simulink model "protocol_mc"  (R2021b)
settings: Solver=FixedStepAuto  StartTime=0.0  StopTime=10.0  RelTol=1e-3
settings Model: Creator=marco  LastModifiedBy=angelo
settings ModelReferenceCC: UpdateModelReferenceTargets=IfOutOfDate
settings ConfigComp: DVTestSuiteOptimization=Auto  DVDetectOutOfBounds=on  DVModelReferenceHarness=on

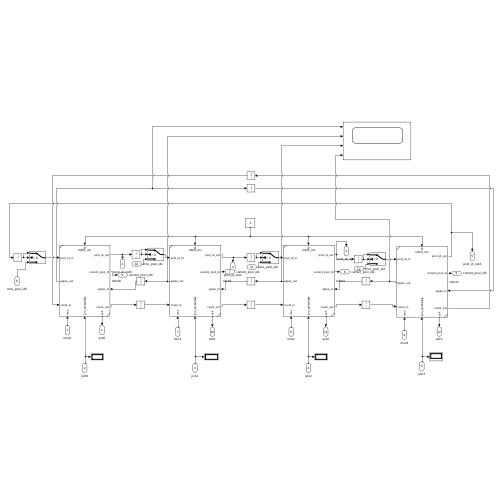
[thumbnail: Simulink's stored preview of the top-level diagram]
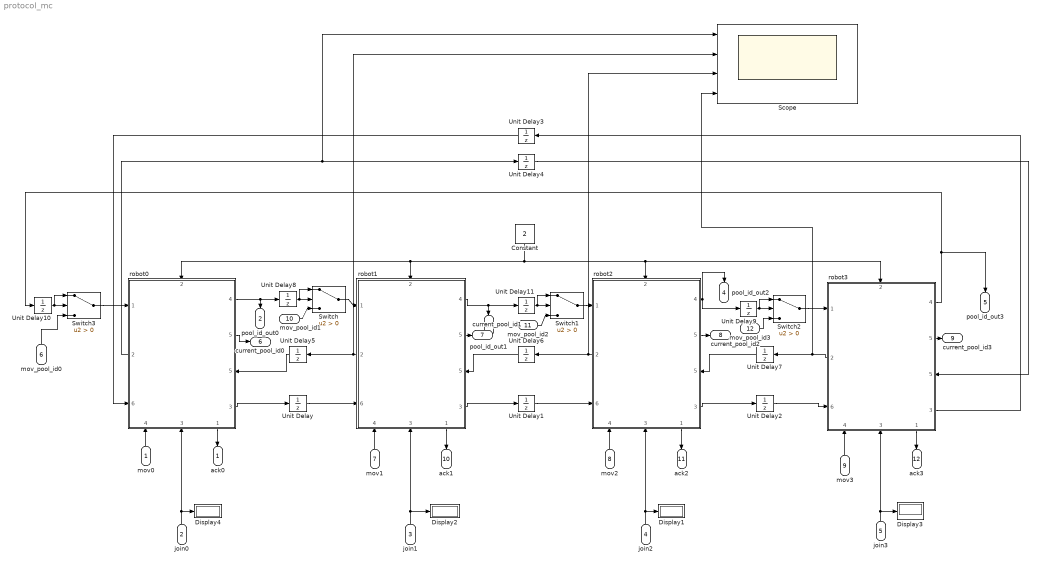
== system protocol_mc ==
  mov0 : Inport
  join0 : Inport  Port=2
  join1 : Inport  Port=3
  join2 : Inport  Port=4
  join3 : Inport  Port=5
  mov_pool_id0 : Inport  Port=6
  mov1 : Inport  Port=7
  mov2 : Inport  Port=8
  mov3 : Inport  Port=9
  mov_pool_id1 : Inport  Port=10
  mov_pool_id2 : Inport  Port=11
  mov_pool_id3 : Inport  Port=12
  Constant : Constant  Value=2
  Display{1..4} (4 alike) : Display
  Scope : Scope  NumInputPorts=4
  Switch{,1..3} (4 alike) : Switch  Criteria=u2 > Threshold
  Unit Delay{,1..11} (12 alike) : UnitDelay  SampleTime=-1  HasFrameUpgradeWarning=on
  robot{0..3} (4 alike) : Subsystem  ReferencedSubsystem=robot_mc
      robot0 settings: PortSchema="{\"entries\":[{\"content\":{\"sides\":[{\"content\":{\"connectorIds\":[\"In1\",\"Out2\",\"In6\"]},\"type\":\"ConnectorPlacement.EquallySpacedRectSide\",\"uuid\":\"c2973ddf-8c1f-4294-82f9-250d4d64bc41\"},{\"content\":{\"connectorIds\":[\"Out4\",\"Out5\",\"In5\",\"Out3\"],\"side\":\"RIGHT\"},\"type\":\"ConnectorPlacement.EquallySpacedRectSide\",\"uuid\":\"34f58778-6b96-4f4c-9fc2-6c1c729063a8\"},{\"content\":{\"connectorIds\":[\"In2\"],\"side\":\"TOP\"},\"type\":\"ConnectorPlacement.EquallySpacedRectSide\",\"uuid\":\"80e910fc-ff47-444b-b672-e337659921ae\"},{\"content\":{\"connectorIds\":[\"In4\",\"In3\",\"Out1\"],\"side\":\"BOTTOM\"},\"type\":\"ConnectorPlacement.EquallySpacedRectSide\",\"uuid\":\"4c5b4a6c-4ee5-43a5-b389-1d5635d4cbda\"}]},\"type\":\"ConnectorPlacement.EquallySpacedConnector\",\"uuid\":\"573bf93a-1f25-4267-812c-06cdd99b033a\"}],\"packageUris\":[\"http://schema.mathworks.com/mf0/Connector/R2020b\"],\"version\":\"1.0\"}"
      robot1 settings: PortSchema="{\"entries\":[{\"content\":{\"sides\":[{\"content\":{\"connectorIds\":[\"In1\",\"Out2\",\"In6\"]},\"type\":\"ConnectorPlacement.EquallySpacedRectSide\",\"uuid\":\"c2973ddf-8c1f-4294-82f9-250d4d64bc41\"},{\"content\":{\"connectorIds\":[\"Out4\",\"Out5\",\"In5\",\"Out3\"],\"side\":\"RIGHT\"},\"type\":\"ConnectorPlacement.EquallySpacedRectSide\",\"uuid\":\"34f58778-6b96-4f4c-9fc2-6c1c729063a8\"},{\"content\":{\"connectorIds\":[\"In2\"],\"side\":\"TOP\"},\"type\":\"ConnectorPlacement.EquallySpacedRectSide\",\"uuid\":\"80e910fc-ff47-444b-b672-e337659921ae\"},{\"content\":{\"connectorIds\":[\"In4\",\"In3\",\"Out1\"],\"side\":\"BOTTOM\"},\"type\":\"ConnectorPlacement.EquallySpacedRectSide\",\"uuid\":\"e4e016b7-b76e-4e62-a0db-89e9df8dea8e\"}]},\"type\":\"ConnectorPlacement.EquallySpacedConnector\",\"uuid\":\"573bf93a-1f25-4267-812c-06cdd99b033a\"}],\"packageUris\":[\"http://schema.mathworks.com/mf0/Connector/R2020b\"],\"version\":\"1.0\"}"
      robot2 settings: PortSchema="{\"entries\":[{\"content\":{\"sides\":[{\"content\":{\"connectorIds\":[\"In1\",\"Out2\",\"In6\"]},\"type\":\"ConnectorPlacement.EquallySpacedRectSide\",\"uuid\":\"c2973ddf-8c1f-4294-82f9-250d4d64bc41\"},{\"content\":{\"connectorIds\":[\"Out4\",\"Out5\",\"In5\",\"Out3\"],\"side\":\"RIGHT\"},\"type\":\"ConnectorPlacement.EquallySpacedRectSide\",\"uuid\":\"34f58778-6b96-4f4c-9fc2-6c1c729063a8\"},{\"content\":{\"connectorIds\":[\"In2\"],\"side\":\"TOP\"},\"type\":\"ConnectorPlacement.EquallySpacedRectSide\",\"uuid\":\"80e910fc-ff47-444b-b672-e337659921ae\"},{\"content\":{\"connectorIds\":[\"In4\",\"In3\",\"Out1\"],\"side\":\"BOTTOM\"},\"type\":\"ConnectorPlacement.EquallySpacedRectSide\",\"uuid\":\"2cd792df-4aad-4f2e-80f9-e48174994b0d\"}]},\"type\":\"ConnectorPlacement.EquallySpacedConnector\",\"uuid\":\"573bf93a-1f25-4267-812c-06cdd99b033a\"}],\"packageUris\":[\"http://schema.mathworks.com/mf0/Connector/R2020b\"],\"version\":\"1.0\"}"
      robot3 settings: PortSchema="{\"entries\":[{\"content\":{\"sides\":[{\"content\":{\"connectorIds\":[\"In1\",\"Out2\",\"In6\"]},\"type\":\"ConnectorPlacement.EquallySpacedRectSide\",\"uuid\":\"c2973ddf-8c1f-4294-82f9-250d4d64bc41\"},{\"content\":{\"connectorIds\":[\"Out4\",\"Out5\",\"In5\",\"Out3\"],\"side\":\"RIGHT\"},\"type\":\"ConnectorPlacement.EquallySpacedRectSide\",\"uuid\":\"34f58778-6b96-4f4c-9fc2-6c1c729063a8\"},{\"content\":{\"connectorIds\":[\"In2\"],\"side\":\"TOP\"},\"type\":\"ConnectorPlacement.EquallySpacedRectSide\",\"uuid\":\"80e910fc-ff47-444b-b672-e337659921ae\"},{\"content\":{\"connectorIds\":[\"In4\",\"In3\",\"Out1\"],\"side\":\"BOTTOM\"},\"type\":\"ConnectorPlacement.EquallySpacedRectSide\",\"uuid\":\"e1d2a9a1-3695-4a7a-a698-108fcecfffe2\"}]},\"type\":\"ConnectorPlacement.EquallySpacedConnector\",\"uuid\":\"573bf93a-1f25-4267-812c-06cdd99b033a\"}],\"packageUris\":[\"http://schema.mathworks.com/mf0/Connector/R2020b\"],\"version\":\"1.0\"}"
  ack0 : Outport
  pool_id_out0 : Outport  Port=2
  pool_id_out1 : Outport  Port=3
  pool_id_out2 : Outport  Port=4
  pool_id_out3 : Outport  Port=5
  current_pool_id0 : Outport  Port=6
  current_pool_id1 : Outport  Port=7
  current_pool_id2 : Outport  Port=8
  current_pool_id3 : Outport  Port=9
  ack1 : Outport  Port=10
  ack2 : Outport  Port=11
  ack3 : Outport  Port=12
  wires:
  robot0/1 -> ack0/1
  robot1/1 -> ack1/1
  robot2/1 -> ack2/1
  robot3/1 -> ack3/1
  robot0/3 -> Unit Delay/1
  robot1/3 -> Unit Delay1/1
  robot2/3 -> Unit Delay2/1
  robot3/3 -> Unit Delay3/1
  robot1/2 -> Unit Delay5/1, Scope/2
  robot2/2 -> Scope/3, Unit Delay6/1
  robot3/2 -> Scope/4, Unit Delay7/1
  robot0/2 -> Scope/1, Unit Delay4/1
  join1/1 -> robot1/3, Display2/1
  join2/1 -> robot2/3, Display1/1
  Unit Delay/1 -> robot1/6
  Unit Delay1/1 -> robot2/6
  Unit Delay2/1 -> robot3/6
  Unit Delay3/1 -> robot0/6
  Unit Delay4/1 -> robot3/5
  Unit Delay5/1 -> robot0/5
  Unit Delay6/1 -> robot1/5
  Unit Delay7/1 -> robot2/5
  join0/1 -> robot0/3, Display4/1
  mov0/1 -> robot0/4
  join3/1 -> robot3/3, Display3/1
  mov2/1 -> robot2/4
  mov3/1 -> robot3/4
  mov1/1 -> robot1/4
  Constant/1 -> robot1/2, robot0/2, robot2/2, robot3/2
  robot0/4 -> Unit Delay8/1, pool_id_out0/1
  robot1/4 -> Unit Delay11/1, pool_id_out1/1
  robot2/4 -> Unit Delay9/1, pool_id_out2/1
  robot3/4 -> Unit Delay10/1, pool_id_out3/1
  robot0/5 -> current_pool_id0/1
  robot1/5 -> current_pool_id1/1
  robot2/5 -> current_pool_id2/1
  robot3/5 -> current_pool_id3/1
  Unit Delay8/1 -> Switch/1, Switch/2
  mov_pool_id1/1 -> Switch/3
  Switch/1 -> robot1/1
  Unit Delay11/1 -> Switch1/1, Switch1/2
  mov_pool_id2/1 -> Switch1/3
  Switch1/1 -> robot2/1
  mov_pool_id3/1 -> Switch2/3
  Unit Delay9/1 -> Switch2/1, Switch2/2
  Switch2/1 -> robot3/1
  mov_pool_id0/1 -> Switch3/3
  Unit Delay10/1 -> Switch3/1, Switch3/2
  Switch3/1 -> robot0/1
